simulink model "forced_msd_test_build"  (Simulink 7.8)
settings: Solver=ode4  StartTime=0.0  StopTime=5  RelTol=1e-3
values from neighbouring files (symbols this model uses):
  outstr = sim_model    [RunCtrlModel.m]    (also in RunCtrlModel_sym.m = model.eqn_str; RunModel.m = model{1}; RunTargetModel.m = model{1})
settings Model: Creator=Kourosh Danai  LastModifiedBy=BionicBill
settings DataIOCC: TimeSaveName=t  OutputSaveName=y
settings DebuggingCC: AlgebraicLoopMsg=none  FcnCallInpInsideContextMsg=Use local settings  StrictBusMsg=Warning
settings SFSimCC: SimParseCustomCode=off

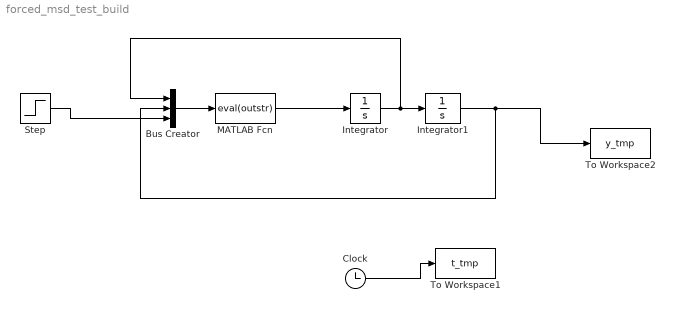
== system forced_msd_test_build ==
  Bus Creator : BusCreator  Inputs=3
  Clock : Clock
  Integrator : Integrator
  Integrator1 : Integrator
  MATLAB Fcn : MATLABFcn  MATLABFcn=eval(outstr)
  Step : Step  Time=0  After=100  SampleTime=.01
  To Workspace1 : ToWorkspace  VariableName=t_tmp  SampleTime=-1  SaveFormat=Array
  To Workspace2 : ToWorkspace  VariableName=y_tmp  SampleTime=-1  SaveFormat=Array
  wires:
  Integrator/1 -> Integrator1/1, Bus Creator/1
  Bus Creator/1 -> MATLAB Fcn/1
  Clock/1 -> To Workspace1/1
  Integrator1/1 -> Bus Creator/2, To Workspace2/1
  MATLAB Fcn/1 -> Integrator/1
  Step/1 -> Bus Creator/3
